simulink model "gm_HA_sys8_vnl"  (R2018a)
settings: Solver=FixedStepDiscrete  StartTime=0.0  StopTime=stopTime  RelTol=1e-3
InitFcn:
  | HA_sys8_init
StopFcn:
  | HA_sys8_freq_response
undefined symbols (not defined in the file or in its folder): dspDeleteFVToolLinkFromMask, FIRBandPass1, FIRBandPass2, FIRBandPass3, FIRBandPass4, FIRDecimator1, FIRDecimator2, FIRDecimator3, FIRDecimator4, FIRInterpolator1, FIRInterpolator2, FIRInterpolator3, FIRInterpolator4, Fs, Gain_B1_left, Gain_B1_right, Gain_B2_left, Gain_B2_right, Gain_B3_left, Gain_B3_right, Gain_B4_left, Gain_B4_right, Gain_left_all, Gain_right_all, gcbh
libraries: hdlsllib x40, dspmlti4 x32, simulink x4, dspsrcs4 x1
(part 3 of 4)

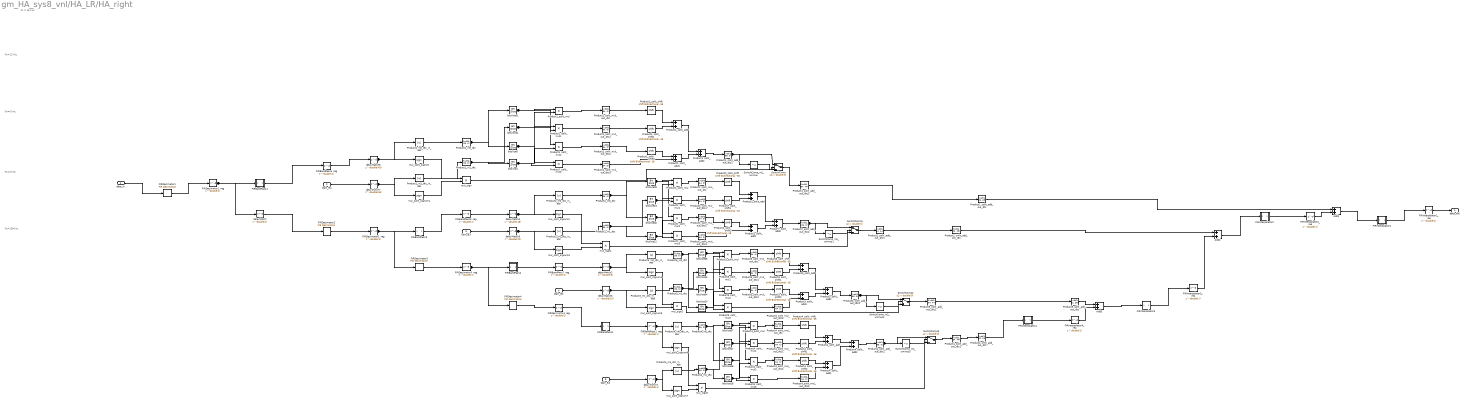
== system gm_HA_sys8_vnl/HA_LR/HA_right ==
  note: Fs = 48 KHz
  note: Fs=12 kHz
  note: Fs=6 kHz
  note: Fs=3 kHz
  note: Fs=1500 Hz
  data_in : Inport  PortDimensions=1  SampleTime=2.08333333333333e-05
  Gain_B4 : Inport  Port=2  OutDataTypeStr=fixdt(1,32,16)  PortDimensions=1  SampleTime=8.33333333333333e-05  LockScale=on
  Gain_B3 : Inport  Port=3  OutDataTypeStr=fixdt(1,32,16)  PortDimensions=1  SampleTime=0.000166666666666667  LockScale=on
  Gain_B2 : Inport  Port=4  OutDataTypeStr=fixdt(1,32,16)  PortDimensions=1  SampleTime=0.000333333333333333  LockScale=on
  Gain_B1 : Inport  Port=5  OutDataTypeStr=fixdt(1,32,16)  PortDimensions=1  SampleTime=0.000666666666666667  LockScale=on
  Add1 : Sum  AccumDataTypeStr=fixdt(1, 33, 28)  OutDataTypeStr=fixdt(1, 33, 28)  SampleTime=8.33333333333333e-05  SaturateOnIntegerOverflow=on
  Add2 : Sum  AccumDataTypeStr=fixdt(1, 33, 28)  OutDataTypeStr=fixdt(1, 33, 28)  SampleTime=0.000166666666666667  SaturateOnIntegerOverflow=on
  Add3 : Sum  AccumDataTypeStr=fixdt(1, 33, 28)  OutDataTypeStr=fixdt(1, 33, 28)  SampleTime=0.000333333333333333  SaturateOnIntegerOverflow=on
  FIRBandPass1 : Subsystem
  FIRBandPass1_reg : Delay  DelayLength=double(1)  InitialCondition=0  InputProcessing=Inherited  SampleTime=0.000666666666666667
  FIRBandPass2 : Subsystem
  FIRBandPass2_reg : Delay  DelayLength=double(1)  InitialCondition=0  InputProcessing=Inherited  SampleTime=0.000333333333333333
  FIRBandPass3 : Subsystem
  FIRBandPass3_reg : Delay  DelayLength=double(1)  InitialCondition=0  InputProcessing=Inherited  SampleTime=0.000166666666666667
  FIRBandPass4 : Subsystem
  FIRBandPass4_reg : Delay  DelayLength=double(1)  InitialCondition=0  InputProcessing=Inherited  SampleTime=8.33333333333333e-05
  FIRDecimator1 : dspmlti4/FIR Decimation  FilterSource=Dialog parameters  h=FIRDecimator1.FIR_coefficients  D=FIRDecimator1.decimation_factor  filtStruct=Direct form  FilterObject=FDECIM  framing=Allow multirate processing  inputOffset=0  outputBufInitCond=0  roundingMode=Floor  overflowMode=on  firstCoeffDataTypeStr=Inherit: Same word length as input  firstCoeffMin=[]  firstCoeffMax=[]  firstCoeffLastDataTypeStr=Inherit: Same word length as input  outputMode=Binary point scaling  outputWordLength=32  outputFracLength=28  outputDataTypeStr=fixdt(1,32,28)  outputMin=[]  outputMax=[]  outputLastDataTypeStr=fixdt(1,32,28)
  FIRDecimator1_reg : Delay  DelayLength=double(1)  InitialCondition=0  InputProcessing=Inherited  SampleTime=8.33333333333333e-05
  FIRDecimator2 : dspmlti4/FIR Decimation  FilterSource=Dialog parameters  h=FIRDecimator2.FIR_coefficients  D=FIRDecimator2.decimation_factor  filtStruct=Direct form  FilterObject=FDECIM  framing=Allow multirate processing  inputOffset=0  outputBufInitCond=0  roundingMode=Floor  overflowMode=on  firstCoeffDataTypeStr=Inherit: Same word length as input  firstCoeffMin=[]  firstCoeffMax=[]  firstCoeffLastDataTypeStr=Inherit: Same word length as input  outputMode=Binary point scaling  outputWordLength=32  outputFracLength=28  outputDataTypeStr=fixdt(1,32,28)  outputMin=[]  outputMax=[]  outputLastDataTypeStr=fixdt(1,32,28)
  FIRDecimator2_reg : Delay  DelayLength=double(1)  InitialCondition=0  InputProcessing=Inherited  SampleTime=0.000166666666666667
  FIRDecimator3 : dspmlti4/FIR Decimation  FilterSource=Dialog parameters  h=FIRDecimator3.FIR_coefficients  D=FIRDecimator3.decimation_factor  filtStruct=Direct form  FilterObject=FDECIM  framing=Allow multirate processing  inputOffset=0  outputBufInitCond=0  roundingMode=Floor  overflowMode=on  firstCoeffDataTypeStr=Inherit: Same word length as input  firstCoeffMin=[]  firstCoeffMax=[]  firstCoeffLastDataTypeStr=Inherit: Same word length as input  outputMode=Binary point scaling  outputWordLength=32  outputFracLength=28  outputDataTypeStr=fixdt(1,32,28)  outputMin=[]  outputMax=[]  outputLastDataTypeStr=fixdt(1,32,28)
  FIRDecimator3_reg : Delay  DelayLength=double(1)  InitialCondition=0  InputProcessing=Inherited  SampleTime=0.000333333333333333
  FIRDecimator4 : dspmlti4/FIR Decimation  FilterSource=Dialog parameters  h=FIRDecimator4.FIR_coefficients  D=FIRDecimator4.decimation_factor  filtStruct=Direct form  FilterObject=FDECIM  framing=Allow multirate processing  inputOffset=0  outputBufInitCond=0  roundingMode=Floor  overflowMode=on  firstCoeffDataTypeStr=Inherit: Same word length as input  firstCoeffMin=[]  firstCoeffMax=[]  firstCoeffLastDataTypeStr=Inherit: Same word length as input  outputMode=Binary point scaling  outputWordLength=32  outputFracLength=28  outputDataTypeStr=fixdt(1,32,28)  outputMin=[]  outputMax=[]  outputLastDataTypeStr=fixdt(1,32,28)
  FIRDecimator4_reg : Delay  DelayLength=double(1)  InitialCondition=0  InputProcessing=Inherited  SampleTime=0.000666666666666667
  FIRInterpolator1 : Subsystem  LoadFcn=dspDeleteFVToolLinkFromMask(gcbh);
      settings: DeleteFcn=dspLinkFVTool2Mask(gcbh,'close')  PreSaveFcn=dspUnlinkFVToolFromMask(gcbh);  PostSaveFcn=dspRestoreLinkFVTool2Mask(gcbh);
      settings: CopyFcn=|
      | ud = get_param(gcbh,'UserData');
      | if isfield(ud,'fvtool')
      |   ud = rmfield(ud,'fvtool');
      |   set_param(gcbh,'UserData',ud);
      | end
      | clear ud;
  FIRInterpolator1_reg : Delay  DelayLength=double(1)  InitialCondition=0  InputProcessing=Inherited  SampleTime=2.08333333333333e-05
  FIRInterpolator2 : Subsystem  LoadFcn=dspDeleteFVToolLinkFromMask(gcbh);
      settings: DeleteFcn=dspLinkFVTool2Mask(gcbh,'close')  PreSaveFcn=dspUnlinkFVToolFromMask(gcbh);  PostSaveFcn=dspRestoreLinkFVTool2Mask(gcbh);
      settings: CopyFcn=|
      | ud = get_param(gcbh,'UserData');
      | if isfield(ud,'fvtool')
      |   ud = rmfield(ud,'fvtool');
      |   set_param(gcbh,'UserData',ud);
      | end
      | clear ud;
  FIRInterpolator2_reg : Delay  DelayLength=double(1)  InitialCondition=0  InputProcessing=Inherited  SampleTime=8.33333333333333e-05
  FIRInterpolator3 : Subsystem  LoadFcn=dspDeleteFVToolLinkFromMask(gcbh);
      settings: DeleteFcn=dspLinkFVTool2Mask(gcbh,'close')  PreSaveFcn=dspUnlinkFVToolFromMask(gcbh);  PostSaveFcn=dspRestoreLinkFVTool2Mask(gcbh);
      settings: CopyFcn=|
      | ud = get_param(gcbh,'UserData');
      | if isfield(ud,'fvtool')
      |   ud = rmfield(ud,'fvtool');
      |   set_param(gcbh,'UserData',ud);
      | end
      | clear ud;
  FIRInterpolator3_reg : Delay  DelayLength=double(1)  InitialCondition=0  InputProcessing=Inherited  SampleTime=0.000166666666666667
  FIRInterpolator4 : Subsystem  LoadFcn=dspDeleteFVToolLinkFromMask(gcbh);
      settings: DeleteFcn=dspLinkFVTool2Mask(gcbh,'close')  PreSaveFcn=dspUnlinkFVToolFromMask(gcbh);  PostSaveFcn=dspRestoreLinkFVTool2Mask(gcbh);
      settings: CopyFcn=|
      | ud = get_param(gcbh,'UserData');
      | if isfield(ud,'fvtool')
      |   ud = rmfield(ud,'fvtool');
      |   set_param(gcbh,'UserData',ud);
      | end
      | clear ud;
  FIRInterpolator4_reg : Delay  DelayLength=double(1)  InitialCondition=0  InputProcessing=Inherited  SampleTime=0.000333333333333333
  Product1_in0_dtc : DataTypeConversion  OutDataTypeStr=fixdt(0, 36, 0)  ConvertRealWorld=Stored Integer (SI)  SampleTime=8.33333333333333e-05
  Product1_in0_dtc_in_abs : Abs  SampleTime=8.33333333333333e-05  OutDataTypeStr=fixdt(0, 32, 28)
  Product1_in1_dtc : DataTypeConversion  OutDataTypeStr=fixdt(0, 36, 0)  ConvertRealWorld=Stored Integer (SI)  SampleTime=8.33333333333333e-05
  Product1_in1_dtc_in_abs : Abs  SampleTime=8.33333333333333e-05  OutDataTypeStr=fixdt(0, 32, 16)
  Product1_split_add : Sum  OutDataTypeStr=fixdt(0, 65, 0)  SampleTime=8.33333333333333e-05
  Product1_split_add1 : Sum  OutDataTypeStr=fixdt(0, 65, 0)  SampleTime=8.33333333333333e-05
  Product1_split_add2 : Sum  OutDataTypeStr=fixdt(0, 66, 0)  SampleTime=8.33333333333333e-05
  Product1_split_add_out_dtc : DataTypeConversion  OutDataTypeStr=fixdt(1, 32, 28)  SampleTime=8.33333333333333e-05  SaturateOnIntegerOverflow=on
  Product1_split_add_out_dtc1 : DataTypeConversion  OutDataTypeStr=fixdt(1, 64, 44)  ConvertRealWorld=Stored Integer (SI)  SampleTime=8.33333333333333e-05
  Product1_split_add_out_dtc2 : DataTypeConversion  OutDataTypeStr=fixdt(1, 66, 0)  SampleTime=8.33333333333333e-05
  Product1_split_mul : Product  Inputs=**  OutDataTypeStr=fixdt(0, 28, 0)  SampleTime=8.33333333333333e-05
  Product1_split_mul1 : Product  Inputs=**  OutDataTypeStr=uint32  SampleTime=8.33333333333333e-05
  Product1_split_mul2 : Product  Inputs=**  OutDataTypeStr=uint32  SampleTime=8.33333333333333e-05
  Product1_split_mul3 : Product  Inputs=**  OutDataTypeStr=fixdt(0, 36, 0)  SampleTime=8.33333333333333e-05
  Product1_split_mul_out_dtc{,1..3} (4 alike) : DataTypeConversion  OutDataTypeStr=fixdt(0, 64, 0)  SampleTime=8.33333333333333e-05
  Product1_split_shift : ArithShift  BitShiftNumber=-36
  Product1_split_shift1 : ArithShift  BitShiftNumber=-18
  Product1_split_shift2 : ArithShift  BitShiftNumber=-18
  Product2_in0_dtc : DataTypeConversion  OutDataTypeStr=fixdt(0, 36, 0)  ConvertRealWorld=Stored Integer (SI)  SampleTime=0.000166666666666667
  Product2_in0_dtc_in_abs : Abs  SampleTime=0.000166666666666667  OutDataTypeStr=fixdt(0, 32, 28)
  Product2_in1_dtc : DataTypeConversion  OutDataTypeStr=fixdt(0, 36, 0)  ConvertRealWorld=Stored Integer (SI)  SampleTime=0.000166666666666667
  Product2_in1_dtc_in_abs : Abs  SampleTime=0.000166666666666667  OutDataTypeStr=fixdt(0, 32, 16)
  Product2_split_add : Sum  OutDataTypeStr=fixdt(0, 65, 0)  SampleTime=0.000166666666666667
  Product2_split_add1 : Sum  OutDataTypeStr=fixdt(0, 65, 0)  SampleTime=0.000166666666666667
  Product2_split_add2 : Sum  OutDataTypeStr=fixdt(0, 66, 0)  SampleTime=0.000166666666666667
  Product2_split_add_out_dtc : DataTypeConversion  OutDataTypeStr=fixdt(1, 32, 28)  SampleTime=0.000166666666666667  SaturateOnIntegerOverflow=on
  Product2_split_add_out_dtc1 : DataTypeConversion  OutDataTypeStr=fixdt(1, 64, 44)  ConvertRealWorld=Stored Integer (SI)  SampleTime=0.000166666666666667
  Product2_split_add_out_dtc2 : DataTypeConversion  OutDataTypeStr=fixdt(1, 66, 0)  SampleTime=0.000166666666666667
  Product2_split_mul : Product  Inputs=**  OutDataTypeStr=fixdt(0, 28, 0)  SampleTime=0.000166666666666667
  Product2_split_mul1 : Product  Inputs=**  OutDataTypeStr=uint32  SampleTime=0.000166666666666667
  Product2_split_mul2 : Product  Inputs=**  OutDataTypeStr=uint32  SampleTime=0.000166666666666667
  Product2_split_mul3 : Product  Inputs=**  OutDataTypeStr=fixdt(0, 36, 0)  SampleTime=0.000166666666666667
  Product2_split_mul_out_dtc{,1..3} (4 alike) : DataTypeConversion  OutDataTypeStr=fixdt(0, 64, 0)  SampleTime=0.000166666666666667
  Product2_split_shift : ArithShift  BitShiftNumber=-36
  Product2_split_shift1 : ArithShift  BitShiftNumber=-18
  Product2_split_shift2 : ArithShift  BitShiftNumber=-18
  Product3_in0_dtc : DataTypeConversion  OutDataTypeStr=fixdt(0, 36, 0)  ConvertRealWorld=Stored Integer (SI)  SampleTime=0.000333333333333333
  Product3_in0_dtc_in_abs : Abs  SampleTime=0.000333333333333333  OutDataTypeStr=fixdt(0, 32, 28)
  Product3_in1_dtc : DataTypeConversion  OutDataTypeStr=fixdt(0, 36, 0)  ConvertRealWorld=Stored Integer (SI)  SampleTime=0.000333333333333333
  Product3_in1_dtc_in_abs : Abs  SampleTime=0.000333333333333333  OutDataTypeStr=fixdt(0, 32, 16)
  Product3_split_add : Sum  OutDataTypeStr=fixdt(0, 65, 0)  SampleTime=0.000333333333333333
  Product3_split_add1 : Sum  OutDataTypeStr=fixdt(0, 65, 0)  SampleTime=0.000333333333333333
  Product3_split_add2 : Sum  OutDataTypeStr=fixdt(0, 66, 0)  SampleTime=0.000333333333333333
  Product3_split_add_out_dtc : DataTypeConversion  OutDataTypeStr=fixdt(1, 32, 28)  SampleTime=0.000333333333333333  SaturateOnIntegerOverflow=on
  Product3_split_add_out_dtc1 : DataTypeConversion  OutDataTypeStr=fixdt(1, 64, 44)  ConvertRealWorld=Stored Integer (SI)  SampleTime=0.000333333333333333
  Product3_split_add_out_dtc2 : DataTypeConversion  OutDataTypeStr=fixdt(1, 66, 0)  SampleTime=0.000333333333333333
  Product3_split_mul : Product  Inputs=**  OutDataTypeStr=fixdt(0, 28, 0)  SampleTime=0.000333333333333333
  Product3_split_mul1 : Product  Inputs=**  OutDataTypeStr=uint32  SampleTime=0.000333333333333333
  Product3_split_mul2 : Product  Inputs=**  OutDataTypeStr=uint32  SampleTime=0.000333333333333333
  Product3_split_mul3 : Product  Inputs=**  OutDataTypeStr=fixdt(0, 36, 0)  SampleTime=0.000333333333333333
  Product3_split_mul_out_dtc{,1..3} (4 alike) : DataTypeConversion  OutDataTypeStr=fixdt(0, 64, 0)  SampleTime=0.000333333333333333
  Product3_split_shift : ArithShift  BitShiftNumber=-36
  Product3_split_shift1 : ArithShift  BitShiftNumber=-18
  Product3_split_shift2 : ArithShift  BitShiftNumber=-18
  Product4_in0_dtc : DataTypeConversion  OutDataTypeStr=fixdt(0, 36, 0)  ConvertRealWorld=Stored Integer (SI)  SampleTime=0.000666666666666667
  Product4_in0_dtc_in_abs : Abs  SampleTime=0.000666666666666667  OutDataTypeStr=fixdt(0, 32, 28)
  Product4_in1_dtc : DataTypeConversion  OutDataTypeStr=fixdt(0, 36, 0)  ConvertRealWorld=Stored Integer (SI)  SampleTime=0.000666666666666667
  Product4_in1_dtc_in_abs : Abs  SampleTime=0.000666666666666667  OutDataTypeStr=fixdt(0, 32, 16)
  Product4_split_add : Sum  OutDataTypeStr=fixdt(0, 65, 0)  SampleTime=0.000666666666666667
  Product4_split_add1 : Sum  OutDataTypeStr=fixdt(0, 65, 0)  SampleTime=0.000666666666666667
  Product4_split_add2 : Sum  OutDataTypeStr=fixdt(0, 66, 0)  SampleTime=0.000666666666666667
  Product4_split_add_out_dtc : DataTypeConversion  OutDataTypeStr=fixdt(1, 32, 28)  SampleTime=0.000666666666666667  SaturateOnIntegerOverflow=on
  Product4_split_add_out_dtc1 : DataTypeConversion  OutDataTypeStr=fixdt(1, 64, 44)  ConvertRealWorld=Stored Integer (SI)  SampleTime=0.000666666666666667
  Product4_split_add_out_dtc2 : DataTypeConversion  OutDataTypeStr=fixdt(1, 66, 0)  SampleTime=0.000666666666666667
  Product4_split_mul : Product  Inputs=**  OutDataTypeStr=fixdt(0, 28, 0)  SampleTime=0.000666666666666667
  Product4_split_mul1 : Product  Inputs=**  OutDataTypeStr=uint32  SampleTime=0.000666666666666667
  Product4_split_mul2 : Product  Inputs=**  OutDataTypeStr=uint32  SampleTime=0.000666666666666667
  Product4_split_mul3 : Product  Inputs=**  OutDataTypeStr=fixdt(0, 36, 0)  SampleTime=0.000666666666666667
  Product4_split_mul_out_dtc{,1..3} (4 alike) : DataTypeConversion  OutDataTypeStr=fixdt(0, 64, 0)  SampleTime=0.000666666666666667
  Product4_split_shift : ArithShift  BitShiftNumber=-36
  Product4_split_shift1 : ArithShift  BitShiftNumber=-18
  Product4_split_shift2 : ArithShift  BitShiftNumber=-18
  SwitchComp : Switch  Criteria=u2 > Threshold  Threshold=double(0)  OutDataTypeStr=fixdt(1, 66, 0)  SampleTime=8.33333333333333e-05
  SwitchComp1 : Switch  Criteria=u2 > Threshold  Threshold=double(0)  OutDataTypeStr=fixdt(1, 66, 0)  SampleTime=0.000166666666666667
  SwitchComp2 : Switch  Criteria=u2 > Threshold  Threshold=double(0)  OutDataTypeStr=fixdt(1, 66, 0)  SampleTime=0.000333333333333333
  SwitchComp3 : Switch  Criteria=u2 > Threshold  Threshold=double(0)  OutDataTypeStr=fixdt(1, 66, 0)  SampleTime=0.000666666666666667
  SwitchComp_in2_uminus : UnaryMinus  SampleTime=8.33333333333333e-05
  SwitchComp_in2_uminus1 : UnaryMinus  SampleTime=0.000166666666666667
  SwitchComp_in2_uminus2 : UnaryMinus  SampleTime=0.000333333333333333
  SwitchComp_in2_uminus3 : UnaryMinus  SampleTime=0.000666666666666667
  bitslice{0..1,12,14,16} (5 alike) : hdlsllib/Logic and Bit Operations/Bit Slice  lidx=double(17)  ridx=double(0)
  bitslice01 : hdlsllib/Logic and Bit Operations/Bit Slice  lidx=double(31)  ridx=double(18)
  bitslice02 : hdlsllib/Logic and Bit Operations/Bit Slice  lidx=double(17)  ridx=double(0)
  bitslice03 : hdlsllib/Logic and Bit Operations/Bit Slice  lidx=double(31)  ridx=double(18)
  bitslice04 : hdlsllib/Logic and Bit Operations/Bit Slice  lidx=double(17)  ridx=double(0)
  bitslice05 : hdlsllib/Logic and Bit Operations/Bit Slice  lidx=double(31)  ridx=double(18)
  bitslice06 : hdlsllib/Logic and Bit Operations/Bit Slice  lidx=double(17)  ridx=double(0)
  bitslice07 : hdlsllib/Logic and Bit Operations/Bit Slice  lidx=double(31)  ridx=double(18)
  bitslice{11,13,15,17} (4 alike) : hdlsllib/Logic and Bit Operations/Bit Slice  lidx=double(31)  ridx=double(18)
  delayMatch : Delay  DelayLength=double(1)  InitialCondition=0  InputProcessing=Inherited  SampleTime=8.33333333333333e-05
  delayMatch1 : Delay  DelayLength=double(4)  InitialCondition=0  InputProcessing=Inherited  SampleTime=0.000666666666666667
  delayMatch2 : Delay  DelayLength=double(6)  InitialCondition=0  InputProcessing=Inherited  SampleTime=0.000333333333333333
  delayMatch3 : Delay  DelayLength=double(10)  InitialCondition=0  InputProcessing=Inherited  SampleTime=0.000333333333333333
  delayMatch4 : Delay  DelayLength=double(18)  InitialCondition=0  InputProcessing=Inherited  SampleTime=0.000166666666666667
  delayMatch5 : Delay  DelayLength=double(22)  InitialCondition=0  InputProcessing=Inherited  SampleTime=0.000166666666666667
  delayMatch6 : Delay  DelayLength=double(43)  InitialCondition=0  InputProcessing=Inherited  SampleTime=8.33333333333333e-05
  delayMatch7 : Delay  DelayLength=double(46)  InitialCondition=0  InputProcessing=Inherited  SampleTime=8.33333333333333e-05
  mul_sign : Product  Inputs=**  OutDataTypeStr=fixdt(1, 2, 0)  SampleTime=8.33333333333333e-05
  mul_sign1 : Product  Inputs=**  OutDataTypeStr=fixdt(1, 2, 0)  SampleTime=0.000166666666666667
  mul_sign2 : Product  Inputs=**  OutDataTypeStr=fixdt(1, 2, 0)  SampleTime=0.000333333333333333
  mul_sign3 : Product  Inputs=**  OutDataTypeStr=fixdt(1, 2, 0)  SampleTime=0.000666666666666667
  mul_split_signum : Signum  SampleTime=8.33333333333333e-05
  mul_split_signum1 : Signum  SampleTime=8.33333333333333e-05
  mul_split_signum2 : Signum  SampleTime=0.000166666666666667
  mul_split_signum3 : Signum  SampleTime=0.000166666666666667
  mul_split_signum4 : Signum  SampleTime=0.000333333333333333
  mul_split_signum5 : Signum  SampleTime=0.000333333333333333
  mul_split_signum6 : Signum  SampleTime=0.000666666666666667
  mul_split_signum7 : Signum  SampleTime=0.000666666666666667
  data_out : Outport
  wires:
  SwitchComp_in2_uminus3/1 -> SwitchComp3/3
  SwitchComp3/1 -> Product4_split_add_out_dtc1/1
  Product4_split_add2/1 -> Product4_split_add_out_dtc2/1
  mul_sign3/1 -> SwitchComp3/2
  mul_split_signum7/1 -> mul_sign3/2
  Product4_in1_dtc_in_abs/1 -> Product4_in1_dtc/1
  mul_split_signum6/1 -> mul_sign3/1
  Product4_in0_dtc_in_abs/1 -> Product4_in0_dtc/1
  Product4_split_add_out_dtc2/1 -> SwitchComp3/1, SwitchComp_in2_uminus3/1
  Product4_split_add_out_dtc1/1 -> Product4_split_add_out_dtc/1
  Product4_split_add1/1 -> Product4_split_add2/2
  Product4_split_add/1 -> Product4_split_add2/1
  Product4_split_mul3/1 -> Product4_split_mul_out_dtc3/1
  Product4_split_mul_out_dtc3/1 -> Product4_split_add1/2
  Product4_split_shift2/1 -> Product4_split_add1/1
  Product4_split_mul2/1 -> Product4_split_mul_out_dtc2/1
  Product4_split_mul_out_dtc2/1 -> Product4_split_shift2/1
  Product4_split_shift1/1 -> Product4_split_add/2
  Product4_split_mul1/1 -> Product4_split_mul_out_dtc1/1
  Product4_split_mul_out_dtc1/1 -> Product4_split_shift1/1
  Product4_split_shift/1 -> Product4_split_add/1
  Product4_split_mul/1 -> Product4_split_mul_out_dtc/1
  Product4_split_mul_out_dtc/1 -> Product4_split_shift/1
  bitslice17/1 -> Product4_split_mul/2, Product4_split_mul1/2
  bitslice16/1 -> Product4_split_mul2/2, Product4_split_mul3/2
  bitslice07/1 -> Product4_split_mul/1, Product4_split_mul2/1
  bitslice06/1 -> Product4_split_mul1/1, Product4_split_mul3/1
  Product4_in1_dtc/1 -> bitslice16/1, bitslice17/1
  Product4_in0_dtc/1 -> bitslice06/1, bitslice07/1
  SwitchComp_in2_uminus2/1 -> SwitchComp2/3
  SwitchComp2/1 -> Product3_split_add_out_dtc1/1
  Product3_split_add2/1 -> Product3_split_add_out_dtc2/1
  mul_sign2/1 -> SwitchComp2/2
  mul_split_signum5/1 -> mul_sign2/2
  Product3_in1_dtc_in_abs/1 -> Product3_in1_dtc/1
  mul_split_signum4/1 -> mul_sign2/1
  Product3_in0_dtc_in_abs/1 -> Product3_in0_dtc/1
  Product3_split_add_out_dtc2/1 -> SwitchComp2/1, SwitchComp_in2_uminus2/1
  Product3_split_add_out_dtc1/1 -> Product3_split_add_out_dtc/1
  Product3_split_add_out_dtc/1 -> Add3/1
  Product3_split_add1/1 -> Product3_split_add2/2
  Product3_split_add/1 -> Product3_split_add2/1
  Product3_split_mul3/1 -> Product3_split_mul_out_dtc3/1
  Product3_split_mul_out_dtc3/1 -> Product3_split_add1/2
  Product3_split_shift2/1 -> Product3_split_add1/1
  Product3_split_mul2/1 -> Product3_split_mul_out_dtc2/1
  Product3_split_mul_out_dtc2/1 -> Product3_split_shift2/1
  Product3_split_shift1/1 -> Product3_split_add/2
  Product3_split_mul1/1 -> Product3_split_mul_out_dtc1/1
  Product3_split_mul_out_dtc1/1 -> Product3_split_shift1/1
  Product3_split_shift/1 -> Product3_split_add/1
  Product3_split_mul/1 -> Product3_split_mul_out_dtc/1
  Product3_split_mul_out_dtc/1 -> Product3_split_shift/1
  bitslice15/1 -> Product3_split_mul/2, Product3_split_mul1/2
  bitslice14/1 -> Product3_split_mul2/2, Product3_split_mul3/2
  bitslice05/1 -> Product3_split_mul/1, Product3_split_mul2/1
  bitslice04/1 -> Product3_split_mul1/1, Product3_split_mul3/1
  Product3_in1_dtc/1 -> bitslice14/1, bitslice15/1
  Product3_in0_dtc/1 -> bitslice04/1, bitslice05/1
  SwitchComp_in2_uminus1/1 -> SwitchComp1/3
  SwitchComp1/1 -> Product2_split_add_out_dtc1/1
  Product2_split_add2/1 -> Product2_split_add_out_dtc2/1
  mul_sign1/1 -> SwitchComp1/2
  mul_split_signum3/1 -> mul_sign1/2
  Product2_in1_dtc_in_abs/1 -> Product2_in1_dtc/1
  mul_split_signum2/1 -> mul_sign1/1
  Product2_in0_dtc_in_abs/1 -> Product2_in0_dtc/1
  Product2_split_add_out_dtc2/1 -> SwitchComp1/1, SwitchComp_in2_uminus1/1
  Product2_split_add_out_dtc1/1 -> Product2_split_add_out_dtc/1
  Product2_split_add_out_dtc/1 -> Add2/1
  Product2_split_add1/1 -> Product2_split_add2/2
  Product2_split_add/1 -> Product2_split_add2/1
  Product2_split_mul3/1 -> Product2_split_mul_out_dtc3/1
  Product2_split_mul_out_dtc3/1 -> Product2_split_add1/2
  Product2_split_shift2/1 -> Product2_split_add1/1
  Product2_split_mul2/1 -> Product2_split_mul_out_dtc2/1
  Product2_split_mul_out_dtc2/1 -> Product2_split_shift2/1
  Product2_split_shift1/1 -> Product2_split_add/2
  Product2_split_mul1/1 -> Product2_split_mul_out_dtc1/1
  Product2_split_mul_out_dtc1/1 -> Product2_split_shift1/1
  Product2_split_shift/1 -> Product2_split_add/1
  Product2_split_mul/1 -> Product2_split_mul_out_dtc/1
  Product2_split_mul_out_dtc/1 -> Product2_split_shift/1
  bitslice13/1 -> Product2_split_mul/2, Product2_split_mul1/2
  bitslice12/1 -> Product2_split_mul2/2, Product2_split_mul3/2
  bitslice03/1 -> Product2_split_mul/1, Product2_split_mul2/1
  bitslice02/1 -> Product2_split_mul1/1, Product2_split_mul3/1
  Product2_in1_dtc/1 -> bitslice12/1, bitslice13/1
  Product2_in0_dtc/1 -> bitslice02/1, bitslice03/1
  SwitchComp_in2_uminus/1 -> SwitchComp/3
  SwitchComp/1 -> Product1_split_add_out_dtc1/1
  Product1_split_add2/1 -> Product1_split_add_out_dtc2/1
  mul_sign/1 -> SwitchComp/2
  mul_split_signum1/1 -> mul_sign/2
  Product1_in1_dtc_in_abs/1 -> Product1_in1_dtc/1
  mul_split_signum/1 -> mul_sign/1
  Product1_in0_dtc_in_abs/1 -> Product1_in0_dtc/1
  Product1_split_add_out_dtc2/1 -> SwitchComp/1, SwitchComp_in2_uminus/1
  Product1_split_add_out_dtc1/1 -> Product1_split_add_out_dtc/1
  Product1_split_add_out_dtc/1 -> Add1/1
  Product1_split_add1/1 -> Product1_split_add2/2
  Product1_split_add/1 -> Product1_split_add2/1
  Product1_split_mul3/1 -> Product1_split_mul_out_dtc3/1
  Product1_split_mul_out_dtc3/1 -> Product1_split_add1/2
  Product1_split_shift2/1 -> Product1_split_add1/1
  Product1_split_mul2/1 -> Product1_split_mul_out_dtc2/1
  Product1_split_mul_out_dtc2/1 -> Product1_split_shift2/1
  Product1_split_shift1/1 -> Product1_split_add/2
  Product1_split_mul1/1 -> Product1_split_mul_out_dtc1/1
  Product1_split_mul_out_dtc1/1 -> Product1_split_shift1/1
  Product1_split_shift/1 -> Product1_split_add/1
  Product1_split_mul/1 -> Product1_split_mul_out_dtc/1
  Product1_split_mul_out_dtc/1 -> Product1_split_shift/1
  bitslice11/1 -> Product1_split_mul/2, Product1_split_mul1/2
  bitslice1/1 -> Product1_split_mul2/2, Product1_split_mul3/2
  bitslice01/1 -> Product1_split_mul/1, Product1_split_mul2/1
  bitslice0/1 -> Product1_split_mul1/1, Product1_split_mul3/1
  Product1_in1_dtc/1 -> bitslice1/1, bitslice11/1
  Product1_in0_dtc/1 -> bitslice0/1, bitslice01/1
  FIRBandPass4_reg/1 -> delayMatch6/1
  FIRBandPass3_reg/1 -> delayMatch4/1
  FIRBandPass2_reg/1 -> delayMatch2/1
  FIRDecimator1_reg/1 -> FIRBandPass4/1(In1), delayMatch/1
  Gain_B1/1 -> delayMatch1/1
  Gain_B2/1 -> delayMatch3/1
  Gain_B3/1 -> delayMatch5/1
  Gain_B4/1 -> delayMatch7/1
  data_in/1 -> FIRDecimator1/1
  Product4_split_add_out_dtc/1 -> FIRInterpolator4/1(In1)
  Add3/1 -> FIRInterpolator3/1(In1)
  Add2/1 -> FIRInterpolator2/1(In1)
  Add1/1 -> FIRInterpolator1/1(In1)
  FIRInterpolator4/1(Out1) -> FIRInterpolator4_reg/1
  FIRInterpolator3/1(Out1) -> FIRInterpolator3_reg/1
  FIRInterpolator2/1(Out1) -> FIRInterpolator2_reg/1
  FIRInterpolator1/1(Out1) -> FIRInterpolator1_reg/1
  FIRDecimator4/1 -> FIRDecimator4_reg/1
  FIRDecimator3/1 -> FIRDecimator3_reg/1
  FIRDecimator2/1 -> FIRDecimator2_reg/1
  FIRDecimator1/1 -> FIRDecimator1_reg/1
  FIRBandPass4/1(Out1) -> FIRBandPass4_reg/1
  FIRBandPass3/1(Out1) -> FIRBandPass3_reg/1
  FIRBandPass2/1(Out1) -> FIRBandPass2_reg/1
  FIRBandPass1/1(Out1) -> FIRBandPass1_reg/1
  FIRInterpolator4_reg/1 -> Add3/2
  FIRInterpolator3_reg/1 -> Add2/2
  FIRInterpolator2_reg/1 -> Add1/2
  FIRInterpolator1_reg/1 -> data_out/1
  FIRDecimator4_reg/1 -> FIRBandPass1/1(In1)
  FIRDecimator3_reg/1 -> FIRDecimator4/1, FIRBandPass2/1(In1)
  FIRDecimator2_reg/1 -> FIRDecimator3/1, FIRBandPass3/1(In1)
  delayMatch/1 -> FIRDecimator2/1
  delayMatch6/1 -> Product1_in0_dtc_in_abs/1, mul_split_signum/1
  delayMatch4/1 -> Product2_in0_dtc_in_abs/1, mul_split_signum2/1
  delayMatch2/1 -> Product3_in0_dtc_in_abs/1, mul_split_signum4/1
  FIRBandPass1_reg/1 -> Product4_in0_dtc_in_abs/1, mul_split_signum6/1
  delayMatch1/1 -> Product4_in1_dtc_in_abs/1, mul_split_signum7/1
  delayMatch3/1 -> Product3_in1_dtc_in_abs/1, mul_split_signum5/1
  delayMatch5/1 -> Product2_in1_dtc_in_abs/1, mul_split_signum3/1
  delayMatch7/1 -> Product1_in1_dtc_in_abs/1, mul_split_signum1/1

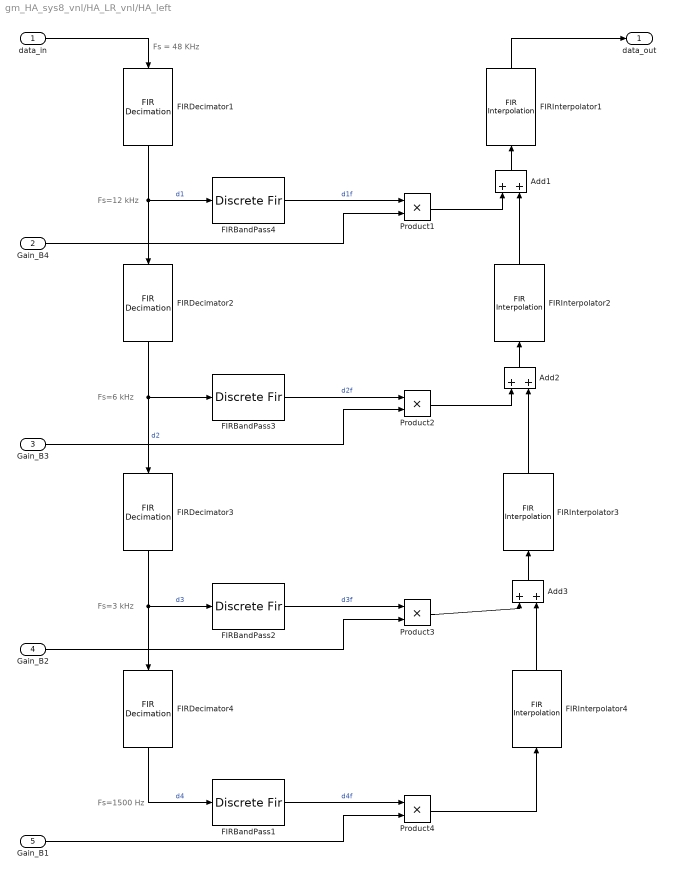
== system gm_HA_sys8_vnl/HA_LR_vnl/HA_left ==
  note: Fs=1500 Hz
  note: Fs=3 kHz
  note: Fs=6 kHz
  note: Fs=12 kHz
  note: Fs = 48 KHz
  data_in : Inport
  Gain_B4 : Inport  Port=2  OutDataTypeStr=fixdt(1,32,16)  LockScale=on
  Gain_B3 : Inport  Port=3  OutDataTypeStr=fixdt(1,32,16)  LockScale=on
  Gain_B2 : Inport  Port=4  OutDataTypeStr=fixdt(1,32,16)  LockScale=on
  Gain_B1 : Inport  Port=5  OutDataTypeStr=fixdt(1,32,16)  LockScale=on
  Add1 : Sum  SaturateOnIntegerOverflow=on
  Add2 : Sum  SaturateOnIntegerOverflow=on
  Add3 : Sum  SaturateOnIntegerOverflow=on
  FIRBandPass1 : DiscreteFir  Coefficients=FIRBandPass1.FIR_coefficients  AccumDataTypeStr=Inherit: Same as product output  OutDataTypeStr=FIRBandPass2.numeric_type  SaturateOnIntegerOverflow=on
  FIRBandPass2 : DiscreteFir  Coefficients=FIRBandPass2.FIR_coefficients  AccumDataTypeStr=Inherit: Same as product output  OutDataTypeStr=FIRBandPass2.numeric_type  SaturateOnIntegerOverflow=on
  FIRBandPass3 : DiscreteFir  Coefficients=FIRBandPass3.FIR_coefficients  AccumDataTypeStr=Inherit: Same as product output  OutDataTypeStr=FIRBandPass2.numeric_type  SaturateOnIntegerOverflow=on
  FIRBandPass4 : DiscreteFir  Coefficients=FIRBandPass4.FIR_coefficients  AccumDataTypeStr=Inherit: Same as product output  SaturateOnIntegerOverflow=on
  FIRDecimator1 : dspmlti4/FIR Decimation  FilterSource=Dialog parameters  h=FIRDecimator1.FIR_coefficients  D=FIRDecimator1.decimation_factor  filtStruct=Direct form  FilterObject=FDECIM  framing=Allow multirate processing  inputOffset=0  outputBufInitCond=0  roundingMode=Floor  overflowMode=on  firstCoeffDataTypeStr=Inherit: Same word length as input  firstCoeffMin=[]  firstCoeffMax=[]  firstCoeffLastDataTypeStr=Inherit: Same word length as input  outputMode=Binary point scaling  outputWordLength=32  outputFracLength=28  outputDataTypeStr=fixdt(1,32,28)  outputMin=[]  outputMax=[]  outputLastDataTypeStr=fixdt(1,32,28)
  FIRDecimator2 : dspmlti4/FIR Decimation  FilterSource=Dialog parameters  h=FIRDecimator2.FIR_coefficients  D=FIRDecimator2.decimation_factor  filtStruct=Direct form  FilterObject=FDECIM  framing=Allow multirate processing  inputOffset=0  outputBufInitCond=0  roundingMode=Floor  overflowMode=on  firstCoeffDataTypeStr=Inherit: Same word length as input  firstCoeffMin=[]  firstCoeffMax=[]  firstCoeffLastDataTypeStr=Inherit: Same word length as input  outputMode=Binary point scaling  outputWordLength=32  outputFracLength=28  outputDataTypeStr=fixdt(1,32,28)  outputMin=[]  outputMax=[]  outputLastDataTypeStr=fixdt(1,32,28)
  FIRDecimator3 : dspmlti4/FIR Decimation  FilterSource=Dialog parameters  h=FIRDecimator3.FIR_coefficients  D=FIRDecimator3.decimation_factor  filtStruct=Direct form  FilterObject=FDECIM  framing=Allow multirate processing  inputOffset=0  outputBufInitCond=0  roundingMode=Floor  overflowMode=on  firstCoeffDataTypeStr=Inherit: Same word length as input  firstCoeffMin=[]  firstCoeffMax=[]  firstCoeffLastDataTypeStr=Inherit: Same word length as input  outputMode=Binary point scaling  outputWordLength=32  outputFracLength=28  outputDataTypeStr=fixdt(1,32,28)  outputMin=[]  outputMax=[]  outputLastDataTypeStr=fixdt(1,32,28)
  FIRDecimator4 : dspmlti4/FIR Decimation  FilterSource=Dialog parameters  h=FIRDecimator4.FIR_coefficients  D=FIRDecimator4.decimation_factor  filtStruct=Direct form  FilterObject=FDECIM  framing=Allow multirate processing  inputOffset=0  outputBufInitCond=0  roundingMode=Floor  overflowMode=on  firstCoeffDataTypeStr=Inherit: Same word length as input  firstCoeffMin=[]  firstCoeffMax=[]  firstCoeffLastDataTypeStr=Inherit: Same word length as input  outputMode=Binary point scaling  outputWordLength=32  outputFracLength=28  outputDataTypeStr=fixdt(1,32,28)  outputMin=[]  outputMax=[]  outputLastDataTypeStr=fixdt(1,32,28)
  FIRInterpolator1 : dspmlti4/FIR Interpolation  FilterSource=Dialog parameters  h=FIRInterpolator1.FIR_coefficients  L=FIRInterpolator1.interpolation_factor  FilterObject=FINTERP  framing=Allow multirate processing  outputBufInitCond=0  roundingMode=Floor  overflowMode=on  firstCoeffDataTypeStr=Inherit: Same word length as input  firstCoeffMin=[]  firstCoeffMax=[]  firstCoeffLastDataTypeStr=Inherit: Same word length as input  outputMode=Binary point scaling  outputWordLength=32  outputFracLength=28  outputDataTypeStr=fixdt(1,32,28)  outputMin=[]  outputMax=[]  outputLastDataTypeStr=fixdt(1,32,28)
      settings: SourceProductName=DSP System Toolbox
  FIRInterpolator2 : dspmlti4/FIR Interpolation  FilterSource=Dialog parameters  h=FIRInterpolator2.FIR_coefficients  L=FIRInterpolator2.interpolation_factor  FilterObject=FINTERP  framing=Allow multirate processing  outputBufInitCond=0  roundingMode=Floor  overflowMode=on  firstCoeffDataTypeStr=Inherit: Same word length as input  firstCoeffMin=[]  firstCoeffMax=[]  firstCoeffLastDataTypeStr=Inherit: Same word length as input  outputMode=Binary point scaling  outputWordLength=32  outputFracLength=28  outputDataTypeStr=fixdt(1,32,28)  outputMin=[]  outputMax=[]  outputLastDataTypeStr=fixdt(1,32,28)
      settings: SourceProductName=DSP System Toolbox
  FIRInterpolator3 : dspmlti4/FIR Interpolation  FilterSource=Dialog parameters  h=FIRInterpolator3.FIR_coefficients  L=FIRInterpolator3.interpolation_factor  FilterObject=FINTERP  framing=Allow multirate processing  outputBufInitCond=0  roundingMode=Floor  overflowMode=on  firstCoeffDataTypeStr=Inherit: Same word length as input  firstCoeffMin=[]  firstCoeffMax=[]  firstCoeffLastDataTypeStr=Inherit: Same word length as input  outputMode=Binary point scaling  outputWordLength=32  outputFracLength=28  outputDataTypeStr=fixdt(1,32,28)  outputMin=[]  outputMax=[]  outputLastDataTypeStr=fixdt(1,32,28)
      settings: SourceProductName=DSP System Toolbox
  FIRInterpolator4 : dspmlti4/FIR Interpolation  FilterSource=Dialog parameters  h=FIRInterpolator4.FIR_coefficients  L=FIRInterpolator4.interpolation_factor  FilterObject=FINTERP  framing=Allow multirate processing  outputBufInitCond=0  roundingMode=Floor  overflowMode=on  firstCoeffDataTypeStr=Inherit: Same word length as input  firstCoeffMin=[]  firstCoeffMax=[]  firstCoeffLastDataTypeStr=Inherit: Same word length as input  outputMode=Binary point scaling  outputWordLength=32  outputFracLength=28  outputDataTypeStr=fixdt(1,32,28)  outputMin=[]  outputMax=[]  outputLastDataTypeStr=fixdt(1,32,28)
      settings: SourceProductName=DSP System Toolbox
  Product{1..4} (4 alike) : Product  OutDataTypeStr=fixdt(1,32,28)  SaturateOnIntegerOverflow=on
  data_out : Outport
  wires:
  Product4/1 -> FIRInterpolator4/1
  FIRInterpolator4/1 -> Add3/2
  Product3/1 -> Add3/1
  Add3/1 -> FIRInterpolator3/1
  FIRDecimator4/1 -> FIRBandPass1/1  "d4"
  Gain_B1/1 -> Product4/2
  FIRBandPass1/1 -> Product4/1  "d4f"
  FIRInterpolator3/1 -> Add2/2
  Product2/1 -> Add2/1
  Add2/1 -> FIRInterpolator2/1
  Gain_B2/1 -> Product3/2
  FIRBandPass2/1 -> Product3/1  "d3f"
  FIRDecimator3/1 -> FIRBandPass2/1, FIRDecimator4/1  "d3"
  FIRInterpolator2/1 -> Add1/2
  Product1/1 -> Add1/1
  Add1/1 -> FIRInterpolator1/1
  FIRDecimator2/1 -> FIRBandPass3/1, FIRDecimator3/1  "d2"
  FIRBandPass3/1 -> Product2/1  "d2f"
  Gain_B3/1 -> Product2/2
  Gain_B4/1 -> Product1/2
  FIRBandPass4/1 -> Product1/1  "d1f"
  FIRDecimator1/1 -> FIRBandPass4/1, FIRDecimator2/1  "d1"
  FIRInterpolator1/1 -> data_out/1
  data_in/1 -> FIRDecimator1/1

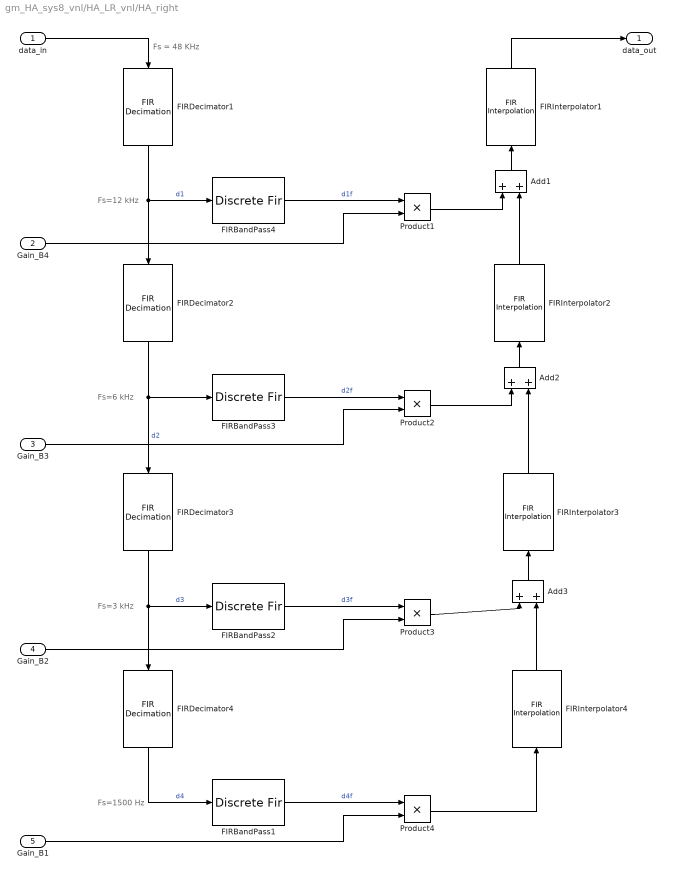
== system gm_HA_sys8_vnl/HA_LR_vnl/HA_right ==
  note: Fs=1500 Hz
  note: Fs=3 kHz
  note: Fs=6 kHz
  note: Fs=12 kHz
  note: Fs = 48 KHz
  data_in : Inport
  Gain_B4 : Inport  Port=2  OutDataTypeStr=fixdt(1,32,16)  LockScale=on
  Gain_B3 : Inport  Port=3  OutDataTypeStr=fixdt(1,32,16)  LockScale=on
  Gain_B2 : Inport  Port=4  OutDataTypeStr=fixdt(1,32,16)  LockScale=on
  Gain_B1 : Inport  Port=5  OutDataTypeStr=fixdt(1,32,16)  LockScale=on
  Add1 : Sum  SaturateOnIntegerOverflow=on
  Add2 : Sum  SaturateOnIntegerOverflow=on
  Add3 : Sum  SaturateOnIntegerOverflow=on
  FIRBandPass1 : DiscreteFir  Coefficients=FIRBandPass1.FIR_coefficients  AccumDataTypeStr=Inherit: Same as product output  OutDataTypeStr=FIRBandPass2.numeric_type  SaturateOnIntegerOverflow=on
  FIRBandPass2 : DiscreteFir  Coefficients=FIRBandPass2.FIR_coefficients  AccumDataTypeStr=Inherit: Same as product output  OutDataTypeStr=FIRBandPass2.numeric_type  SaturateOnIntegerOverflow=on
  FIRBandPass3 : DiscreteFir  Coefficients=FIRBandPass3.FIR_coefficients  AccumDataTypeStr=Inherit: Same as product output  OutDataTypeStr=FIRBandPass2.numeric_type  SaturateOnIntegerOverflow=on
  FIRBandPass4 : DiscreteFir  Coefficients=FIRBandPass4.FIR_coefficients  AccumDataTypeStr=Inherit: Same as product output  SaturateOnIntegerOverflow=on
  FIRDecimator1 : dspmlti4/FIR Decimation  FilterSource=Dialog parameters  h=FIRDecimator1.FIR_coefficients  D=FIRDecimator1.decimation_factor  filtStruct=Direct form  FilterObject=FDECIM  framing=Allow multirate processing  inputOffset=0  outputBufInitCond=0  roundingMode=Floor  overflowMode=on  firstCoeffDataTypeStr=Inherit: Same word length as input  firstCoeffMin=[]  firstCoeffMax=[]  firstCoeffLastDataTypeStr=Inherit: Same word length as input  outputMode=Binary point scaling  outputWordLength=32  outputFracLength=28  outputDataTypeStr=fixdt(1,32,28)  outputMin=[]  outputMax=[]  outputLastDataTypeStr=fixdt(1,32,28)
  FIRDecimator2 : dspmlti4/FIR Decimation  FilterSource=Dialog parameters  h=FIRDecimator2.FIR_coefficients  D=FIRDecimator2.decimation_factor  filtStruct=Direct form  FilterObject=FDECIM  framing=Allow multirate processing  inputOffset=0  outputBufInitCond=0  roundingMode=Floor  overflowMode=on  firstCoeffDataTypeStr=Inherit: Same word length as input  firstCoeffMin=[]  firstCoeffMax=[]  firstCoeffLastDataTypeStr=Inherit: Same word length as input  outputMode=Binary point scaling  outputWordLength=32  outputFracLength=28  outputDataTypeStr=fixdt(1,32,28)  outputMin=[]  outputMax=[]  outputLastDataTypeStr=fixdt(1,32,28)
  FIRDecimator3 : dspmlti4/FIR Decimation  FilterSource=Dialog parameters  h=FIRDecimator3.FIR_coefficients  D=FIRDecimator3.decimation_factor  filtStruct=Direct form  FilterObject=FDECIM  framing=Allow multirate processing  inputOffset=0  outputBufInitCond=0  roundingMode=Floor  overflowMode=on  firstCoeffDataTypeStr=Inherit: Same word length as input  firstCoeffMin=[]  firstCoeffMax=[]  firstCoeffLastDataTypeStr=Inherit: Same word length as input  outputMode=Binary point scaling  outputWordLength=32  outputFracLength=28  outputDataTypeStr=fixdt(1,32,28)  outputMin=[]  outputMax=[]  outputLastDataTypeStr=fixdt(1,32,28)
  FIRDecimator4 : dspmlti4/FIR Decimation  FilterSource=Dialog parameters  h=FIRDecimator4.FIR_coefficients  D=FIRDecimator4.decimation_factor  filtStruct=Direct form  FilterObject=FDECIM  framing=Allow multirate processing  inputOffset=0  outputBufInitCond=0  roundingMode=Floor  overflowMode=on  firstCoeffDataTypeStr=Inherit: Same word length as input  firstCoeffMin=[]  firstCoeffMax=[]  firstCoeffLastDataTypeStr=Inherit: Same word length as input  outputMode=Binary point scaling  outputWordLength=32  outputFracLength=28  outputDataTypeStr=fixdt(1,32,28)  outputMin=[]  outputMax=[]  outputLastDataTypeStr=fixdt(1,32,28)
  FIRInterpolator1 : dspmlti4/FIR Interpolation  FilterSource=Dialog parameters  h=FIRInterpolator1.FIR_coefficients  L=FIRInterpolator1.interpolation_factor  FilterObject=FINTERP  framing=Allow multirate processing  outputBufInitCond=0  roundingMode=Floor  overflowMode=on  firstCoeffDataTypeStr=Inherit: Same word length as input  firstCoeffMin=[]  firstCoeffMax=[]  firstCoeffLastDataTypeStr=Inherit: Same word length as input  outputMode=Binary point scaling  outputWordLength=32  outputFracLength=28  outputDataTypeStr=fixdt(1,32,28)  outputMin=[]  outputMax=[]  outputLastDataTypeStr=fixdt(1,32,28)
      settings: SourceProductName=DSP System Toolbox
  FIRInterpolator2 : dspmlti4/FIR Interpolation  FilterSource=Dialog parameters  h=FIRInterpolator2.FIR_coefficients  L=FIRInterpolator2.interpolation_factor  FilterObject=FINTERP  framing=Allow multirate processing  outputBufInitCond=0  roundingMode=Floor  overflowMode=on  firstCoeffDataTypeStr=Inherit: Same word length as input  firstCoeffMin=[]  firstCoeffMax=[]  firstCoeffLastDataTypeStr=Inherit: Same word length as input  outputMode=Binary point scaling  outputWordLength=32  outputFracLength=28  outputDataTypeStr=fixdt(1,32,28)  outputMin=[]  outputMax=[]  outputLastDataTypeStr=fixdt(1,32,28)
      settings: SourceProductName=DSP System Toolbox
  FIRInterpolator3 : dspmlti4/FIR Interpolation  FilterSource=Dialog parameters  h=FIRInterpolator3.FIR_coefficients  L=FIRInterpolator3.interpolation_factor  FilterObject=FINTERP  framing=Allow multirate processing  outputBufInitCond=0  roundingMode=Floor  overflowMode=on  firstCoeffDataTypeStr=Inherit: Same word length as input  firstCoeffMin=[]  firstCoeffMax=[]  firstCoeffLastDataTypeStr=Inherit: Same word length as input  outputMode=Binary point scaling  outputWordLength=32  outputFracLength=28  outputDataTypeStr=fixdt(1,32,28)  outputMin=[]  outputMax=[]  outputLastDataTypeStr=fixdt(1,32,28)
      settings: SourceProductName=DSP System Toolbox
  FIRInterpolator4 : dspmlti4/FIR Interpolation  FilterSource=Dialog parameters  h=FIRInterpolator4.FIR_coefficients  L=FIRInterpolator4.interpolation_factor  FilterObject=FINTERP  framing=Allow multirate processing  outputBufInitCond=0  roundingMode=Floor  overflowMode=on  firstCoeffDataTypeStr=Inherit: Same word length as input  firstCoeffMin=[]  firstCoeffMax=[]  firstCoeffLastDataTypeStr=Inherit: Same word length as input  outputMode=Binary point scaling  outputWordLength=32  outputFracLength=28  outputDataTypeStr=fixdt(1,32,28)  outputMin=[]  outputMax=[]  outputLastDataTypeStr=fixdt(1,32,28)
      settings: SourceProductName=DSP System Toolbox
  Product{1..4} (4 alike) : Product  OutDataTypeStr=fixdt(1,32,28)  SaturateOnIntegerOverflow=on
  data_out : Outport
  wires:
  Product4/1 -> FIRInterpolator4/1
  FIRInterpolator4/1 -> Add3/2
  Product3/1 -> Add3/1
  Add3/1 -> FIRInterpolator3/1
  FIRDecimator4/1 -> FIRBandPass1/1  "d4"
  Gain_B1/1 -> Product4/2
  FIRBandPass1/1 -> Product4/1  "d4f"
  FIRInterpolator3/1 -> Add2/2
  Product2/1 -> Add2/1
  Add2/1 -> FIRInterpolator2/1
  Gain_B2/1 -> Product3/2
  FIRBandPass2/1 -> Product3/1  "d3f"
  FIRDecimator3/1 -> FIRBandPass2/1, FIRDecimator4/1  "d3"
  FIRInterpolator2/1 -> Add1/2
  Product1/1 -> Add1/1
  Add1/1 -> FIRInterpolator1/1
  FIRDecimator2/1 -> FIRBandPass3/1, FIRDecimator3/1  "d2"
  FIRBandPass3/1 -> Product2/1  "d2f"
  Gain_B3/1 -> Product2/2
  Gain_B4/1 -> Product1/2
  FIRBandPass4/1 -> Product1/1  "d1f"
  FIRDecimator1/1 -> FIRBandPass4/1, FIRDecimator2/1  "d1"
  FIRInterpolator1/1 -> data_out/1
  data_in/1 -> FIRDecimator1/1

== system gm_HA_sys8_vnl/HA_LR/HA_left/FIRBandPass1 ==
  In1 : Inport
  FIRBandPass1 : DiscreteFir  Coefficients=FIRBandPass1.FIR_coefficients  CoefDataTypeStr=fixdt(1,32,32)  ProductDataTypeStr=fixdt(1,63,60)  AccumDataTypeStr=fixdt(1,65,60)  OutDataTypeStr=fixdt(1,32,28)  SaturateOnIntegerOverflow=on
  FIRBandPass1_GenDelay1 : Delay  DelayLength=1  InputProcessing=Inherited
  Out1 : Outport
  wires:
  FIRBandPass1_GenDelay1/1 -> Out1/1
  FIRBandPass1/1 -> FIRBandPass1_GenDelay1/1
  In1/1 -> FIRBandPass1/1

== system gm_HA_sys8_vnl/HA_LR/HA_left/FIRBandPass2 ==
  In1 : Inport
  FIRBandPass2 : DiscreteFir  Coefficients=FIRBandPass2.FIR_coefficients  CoefDataTypeStr=fixdt(1,32,32)  ProductDataTypeStr=fixdt(1,63,60)  AccumDataTypeStr=fixdt(1,65,60)  OutDataTypeStr=fixdt(1,32,28)  SaturateOnIntegerOverflow=on
  FIRBandPass2_GenDelay1 : Delay  DelayLength=1  InputProcessing=Inherited
  Out1 : Outport
  wires:
  FIRBandPass2_GenDelay1/1 -> Out1/1
  FIRBandPass2/1 -> FIRBandPass2_GenDelay1/1
  In1/1 -> FIRBandPass2/1

== system gm_HA_sys8_vnl/HA_LR/HA_left/FIRBandPass3 ==
  In1 : Inport
  FIRBandPass3 : DiscreteFir  Coefficients=FIRBandPass3.FIR_coefficients  CoefDataTypeStr=fixdt(1,32,32)  ProductDataTypeStr=fixdt(1,63,60)  AccumDataTypeStr=fixdt(1,65,60)  OutDataTypeStr=fixdt(1,32,28)  SaturateOnIntegerOverflow=on
  FIRBandPass3_GenDelay1 : Delay  DelayLength=1  InputProcessing=Inherited
  Out1 : Outport
  wires:
  FIRBandPass3_GenDelay1/1 -> Out1/1
  FIRBandPass3/1 -> FIRBandPass3_GenDelay1/1
  In1/1 -> FIRBandPass3/1

== system gm_HA_sys8_vnl/HA_LR/HA_left/FIRBandPass4 ==
  In1 : Inport
  FIRBandPass4 : DiscreteFir  Coefficients=FIRBandPass4.FIR_coefficients  CoefDataTypeStr=fixdt(1,32,32)  ProductDataTypeStr=fixdt(1,63,60)  AccumDataTypeStr=fixdt(1,65,60)  OutDataTypeStr=fixdt(1,32,28)  SaturateOnIntegerOverflow=on
  FIRBandPass4_GenDelay1 : Delay  DelayLength=1  InputProcessing=Inherited
  Out1 : Outport
  wires:
  FIRBandPass4_GenDelay1/1 -> Out1/1
  FIRBandPass4/1 -> FIRBandPass4_GenDelay1/1
  In1/1 -> FIRBandPass4/1

== system gm_HA_sys8_vnl/HA_LR/HA_left/FIRInterpolator1 ==
  In1 : Inport
  FIRInterpolator1 : dspmlti4/FIR Interpolation  FilterSource=Dialog parameters  h=FIRInterpolator1.FIR_coefficients  L=FIRInterpolator1.interpolation_factor  FilterObject=FINTERP  framing=Allow multirate processing  outputBufInitCond=0  roundingMode=Floor  overflowMode=on  firstCoeffDataTypeStr=Inherit: Same word length as input  firstCoeffMin=[]  firstCoeffMax=[]  firstCoeffLastDataTypeStr=Inherit: Same word length as input  outputMode=Binary point scaling  outputWordLength=32  outputFracLength=28  outputDataTypeStr=fixdt(1,32,28)  outputMin=[]  outputMax=[]  outputLastDataTypeStr=fixdt(1,32,28)
      settings: SourceProductName=DSP System Toolbox
  FIRInterpolator1_GenDelay1 : Delay  DelayLength=1  InputProcessing=Inherited
  Out1 : Outport
  wires:
  FIRInterpolator1_GenDelay1/1 -> Out1/1
  FIRInterpolator1/1 -> FIRInterpolator1_GenDelay1/1
  In1/1 -> FIRInterpolator1/1

== system gm_HA_sys8_vnl/HA_LR/HA_left/FIRInterpolator2 ==
  In1 : Inport
  FIRInterpolator2 : dspmlti4/FIR Interpolation  FilterSource=Dialog parameters  h=FIRInterpolator2.FIR_coefficients  L=FIRInterpolator2.interpolation_factor  FilterObject=FINTERP  framing=Allow multirate processing  outputBufInitCond=0  roundingMode=Floor  overflowMode=on  firstCoeffDataTypeStr=Inherit: Same word length as input  firstCoeffMin=[]  firstCoeffMax=[]  firstCoeffLastDataTypeStr=Inherit: Same word length as input  outputMode=Binary point scaling  outputWordLength=32  outputFracLength=28  outputDataTypeStr=fixdt(1,32,28)  outputMin=[]  outputMax=[]  outputLastDataTypeStr=fixdt(1,32,28)
      settings: SourceProductName=DSP System Toolbox
  FIRInterpolator2_GenDelay1 : Delay  DelayLength=1  InputProcessing=Inherited
  Out1 : Outport
  wires:
  FIRInterpolator2_GenDelay1/1 -> Out1/1
  FIRInterpolator2/1 -> FIRInterpolator2_GenDelay1/1
  In1/1 -> FIRInterpolator2/1

== system gm_HA_sys8_vnl/HA_LR/HA_left/FIRInterpolator3 ==
  In1 : Inport
  FIRInterpolator3 : dspmlti4/FIR Interpolation  FilterSource=Dialog parameters  h=FIRInterpolator3.FIR_coefficients  L=FIRInterpolator3.interpolation_factor  FilterObject=FINTERP  framing=Allow multirate processing  outputBufInitCond=0  roundingMode=Floor  overflowMode=on  firstCoeffDataTypeStr=Inherit: Same word length as input  firstCoeffMin=[]  firstCoeffMax=[]  firstCoeffLastDataTypeStr=Inherit: Same word length as input  outputMode=Binary point scaling  outputWordLength=32  outputFracLength=28  outputDataTypeStr=fixdt(1,32,28)  outputMin=[]  outputMax=[]  outputLastDataTypeStr=fixdt(1,32,28)
      settings: SourceProductName=DSP System Toolbox
  FIRInterpolator3_GenDelay1 : Delay  DelayLength=1  InputProcessing=Inherited
  Out1 : Outport
  wires:
  FIRInterpolator3_GenDelay1/1 -> Out1/1
  FIRInterpolator3/1 -> FIRInterpolator3_GenDelay1/1
  In1/1 -> FIRInterpolator3/1

== system gm_HA_sys8_vnl/HA_LR/HA_left/FIRInterpolator4 ==
  In1 : Inport
  FIRInterpolator4 : dspmlti4/FIR Interpolation  FilterSource=Dialog parameters  h=FIRInterpolator4.FIR_coefficients  L=FIRInterpolator4.interpolation_factor  FilterObject=FINTERP  framing=Allow multirate processing  outputBufInitCond=0  roundingMode=Floor  overflowMode=on  firstCoeffDataTypeStr=Inherit: Same word length as input  firstCoeffMin=[]  firstCoeffMax=[]  firstCoeffLastDataTypeStr=Inherit: Same word length as input  outputMode=Binary point scaling  outputWordLength=32  outputFracLength=28  outputDataTypeStr=fixdt(1,32,28)  outputMin=[]  outputMax=[]  outputLastDataTypeStr=fixdt(1,32,28)
      settings: SourceProductName=DSP System Toolbox
  FIRInterpolator4_GenDelay1 : Delay  DelayLength=1  InputProcessing=Inherited
  Out1 : Outport
  wires:
  FIRInterpolator4_GenDelay1/1 -> Out1/1
  FIRInterpolator4/1 -> FIRInterpolator4_GenDelay1/1
  In1/1 -> FIRInterpolator4/1

== system gm_HA_sys8_vnl/HA_LR/HA_right/FIRBandPass1 ==
  In1 : Inport
  FIRBandPass1 : DiscreteFir  Coefficients=FIRBandPass1.FIR_coefficients  CoefDataTypeStr=fixdt(1,32,32)  ProductDataTypeStr=fixdt(1,63,60)  AccumDataTypeStr=fixdt(1,65,60)  OutDataTypeStr=fixdt(1,32,28)  SaturateOnIntegerOverflow=on
  FIRBandPass1_GenDelay1 : Delay  DelayLength=1  InputProcessing=Inherited
  Out1 : Outport
  wires:
  FIRBandPass1_GenDelay1/1 -> Out1/1
  FIRBandPass1/1 -> FIRBandPass1_GenDelay1/1
  In1/1 -> FIRBandPass1/1

== system gm_HA_sys8_vnl/HA_LR/HA_right/FIRBandPass2 ==
  In1 : Inport
  FIRBandPass2 : DiscreteFir  Coefficients=FIRBandPass2.FIR_coefficients  CoefDataTypeStr=fixdt(1,32,32)  ProductDataTypeStr=fixdt(1,63,60)  AccumDataTypeStr=fixdt(1,65,60)  OutDataTypeStr=fixdt(1,32,28)  SaturateOnIntegerOverflow=on
  FIRBandPass2_GenDelay1 : Delay  DelayLength=1  InputProcessing=Inherited
  Out1 : Outport
  wires:
  FIRBandPass2_GenDelay1/1 -> Out1/1
  FIRBandPass2/1 -> FIRBandPass2_GenDelay1/1
  In1/1 -> FIRBandPass2/1

== system gm_HA_sys8_vnl/HA_LR/HA_right/FIRBandPass3 ==
  In1 : Inport
  FIRBandPass3 : DiscreteFir  Coefficients=FIRBandPass3.FIR_coefficients  CoefDataTypeStr=fixdt(1,32,32)  ProductDataTypeStr=fixdt(1,63,60)  AccumDataTypeStr=fixdt(1,65,60)  OutDataTypeStr=fixdt(1,32,28)  SaturateOnIntegerOverflow=on
  FIRBandPass3_GenDelay1 : Delay  DelayLength=1  InputProcessing=Inherited
  Out1 : Outport
  wires:
  FIRBandPass3_GenDelay1/1 -> Out1/1
  FIRBandPass3/1 -> FIRBandPass3_GenDelay1/1
  In1/1 -> FIRBandPass3/1

== system gm_HA_sys8_vnl/HA_LR/HA_right/FIRBandPass4 ==
  In1 : Inport
  FIRBandPass4 : DiscreteFir  Coefficients=FIRBandPass4.FIR_coefficients  CoefDataTypeStr=fixdt(1,32,32)  ProductDataTypeStr=fixdt(1,63,60)  AccumDataTypeStr=fixdt(1,65,60)  OutDataTypeStr=fixdt(1,32,28)  SaturateOnIntegerOverflow=on
  FIRBandPass4_GenDelay1 : Delay  DelayLength=1  InputProcessing=Inherited
  Out1 : Outport
  wires:
  FIRBandPass4_GenDelay1/1 -> Out1/1
  FIRBandPass4/1 -> FIRBandPass4_GenDelay1/1
  In1/1 -> FIRBandPass4/1
